simulink library "seb"  (Simulink 8.1)
settings: Solver=ode1  StartTime=0.0  StopTime=Inf  FixedStep=0.001  RelTol=1e-3
PostLoadFcn:
  | , if any(exist('dsrtsu_mdlpostloadfcn', 'file') == [2, 3, 6]), try dsrtsu_mdlpostloadfcn('Execute', bdroot); catch fprintf('Error in PostLoadFcn (dsrtsu_mdlpostloadfcn) for model "%s":\n %s\n', bdroot, lasterr); end, end,
undefined symbols (not defined in the file or in its folder): ENUM_AEBSTATE_AUTOBRAKING, ENUM_AEBSTATE_BRAKEASSIST, ENUM_AEBSTATE_DISABLED, ENUM_AEBSTATE_OPERATIONAL, ENUM_AEBSTATE_PREBRAKING, ENUM_AEBSTATE_STANDBY, ENUM_HMISTATE_ACTIVE, ENUM_HMISTATE_DISABLED, ENUM_HMISTATE_STANDBY, FALSE, TRUE, ZERO_FLOAT
settings Model: DSRTSU_INTERNAL_RTI_VER=450  DSRTSU_INTERNAL_RTI_TYPE=rti1401  RTICANMMDATA=struct('GeneralSetupData',struct('modelroot','D:\Soichi\SVNDATA\IDIADA_ADAS\trunk\AdasDragon\software\sw_development\arch\app\aeb','generalsettings',struct('filesettings',struct('destfolder',struct('Name','RTICANMM_FILES','Check',1),'buildfolder',struct('Name','.','Check',1),'AbsDestfolder',struct('Name','D:\Soichi\SVNDATA\IDIADA_ADAS\trunk\AdasDragon\software\sw_development\arch\app\aeb\RTICANMM_FILES'),'AbsBuildfolder',struct('Name','D:\Soichi\SVNDATA\IDIADA_ADAS\trunk\AdasDragon\software\sw_development\arch\app\aeb'))),'options',struct('addpaths',1,'rmpaths',1,'addtrcexclusion',logical(1),'cannavigator',struct('checkmonitoring',0),'show_usrtrc',0,'use_usrtrc',0),'advanced',struct('options',[1 1 1 1 1 1 1 1 1 1 1 1 1 1 1 1 1 1 1 1 1 1 1 1 1 1 1 1 1 1 1 1 1 1 1 1 1 1 1 1 1 1 1 1 1 1 1 1 1 1 1 1 1 1 1 1 1 1 1 1 1 1 1 1 1 1 1 1 1 1 1 1 1 1 1 1 1 1 1 1 1 1 1 1 1 1 1 1 1 1 1 1 1 1 1 1 1 1 1 1]),'MPSetup',{{}},'modelname','seb','block','seb'))  DSRTSU_INTERNAL_RTIFPGA=40  Creator=tescamilla  LastModifiedBy=AT015411

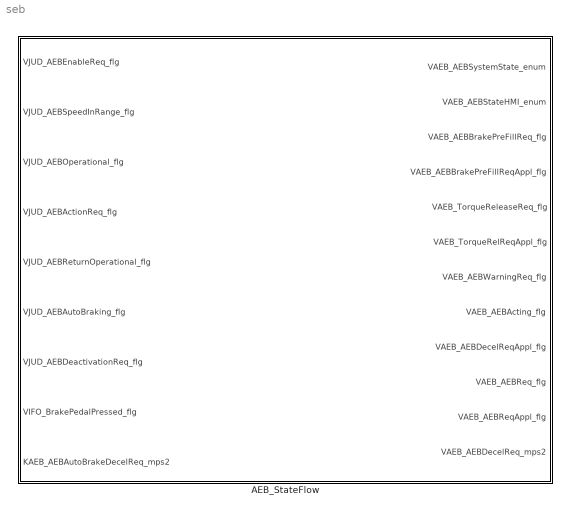
== system seb ==
  AEB_StateFlow : Stateflow chart  TreatAsAtomicUnit=on

== stateflow chart AEB_StateFlow ==
  state DISABLED
    en:
    VAEB_AEBSystemState_enum= ENUM_AEBSTATE_DISABLED;
    VAEB_AEBStateHMI_enum = ENUM_HMISTATE_DISABLED;
    VAEB_AEBWarningReq_flg = FALSE;
    VAEB_AEBActing_flg = FALSE;
    VAEB_TorqueReleaseReq_flg = FALSE;
    VAEB_TorqueRelReqAppl_flg = FALSE;
    VAEB_AEBBrakePreFillReq_flg = FALSE;
    VAEB_AEBBrakePreFillReqAppl_flg = FALSE;
    VAEB_AEBDecelReq_mps2 = ZERO_FLOAT;
    VAEB_AEBDecelReqAppl_flg = FALSE;
    VAEB_AEBReq_flg = FALSE;
    VAEB_AEBReqAppl_flg = FALSE;
  state ENABLED
    state STANDBY
      en:
      VAEB_AEBSystemState_enum = ENUM_AEBSTATE_STANDBY;
      VAEB_AEBStateHMI_enum = ENUM_HMISTATE_STANDBY;
    state ACTIVE
      state OPERATIONAL
        en:
        VAEB_AEBSystemState_enum = ENUM_AEBSTATE_OPERATIONAL;
        VAEB_AEBStateHMI_enum = ENUM_HMISTATE_STANDBY;
      state ACTING
        en:
        VAEB_AEBStateHMI_enum = ENUM_HMISTATE_ACTIVE;
        VAEB_AEBWarningReq_flg = TRUE;
        VAEB_AEBActing_flg=TRUE;
        VAEB_TorqueReleaseReq_flg = TRUE;
        VAEB_TorqueRelReqAppl_flg = TRUE;
        ex:
        VAEB_AEBWarningReq_flg = FALSE;
        VAEB_AEBActing_flg = FALSE;
        VAEB_TorqueReleaseReq_flg = FALSE;
        VAEB_TorqueRelReqAppl_flg = FALSE;
        state PREBRAKING
          en:
          VAEB_AEBSystemState_enum = ENUM_AEBSTATE_PREBRAKING;
          VAEB_AEBBrakePreFillReq_flg = TRUE;
          VAEB_AEBBrakePreFillReqAppl_flg = TRUE;
          ex:
          VAEB_AEBBrakePreFillReq_flg = FALSE;
          VAEB_AEBBrakePreFillReqAppl_flg = FALSE;
        state AUTO_BRAKING
          en:
          VAEB_AEBSystemState_enum = ENUM_AEBSTATE_AUTOBRAKING;
          VAEB_AEBDecelReqAppl_flg = TRUE;
          VAEB_AEBDecelReq_mps2 = KAEB_AEBAutoBrakeDecelReq_mps2;
          ex:
          VAEB_AEBDecelReqAppl_flg = FALSE;
          VAEB_AEBDecelReq_mps2 = ZERO_FLOAT;
        state BRAKE_ASSIST
          en:
          VAEB_AEBSystemState_enum = ENUM_AEBSTATE_BRAKEASSIST;
          VAEB_AEBReq_flg = TRUE;
          VAEB_AEBReqAppl_flg = TRUE;
          ex:
          VAEB_AEBReq_flg = FALSE;
          VAEB_AEBReqAppl_flg = FALSE;
        (default) -> PREBRAKING
        AUTO_BRAKING -> BRAKE_ASSIST : [VIFO_BrakePedalPressed_flg == TRUE]
        PREBRAKING -> AUTO_BRAKING [order 1] : [VJUD_AEBAutoBraking_flg==TRUE]
        PREBRAKING -> (junction 19) [order 2]
        (junction 20) -> BRAKE_ASSIST
        (junction 19) -> (junction 20) : [VIFO_BrakePedalPressed_flg == TRUE]
      (default) -> OPERATIONAL
      OPERATIONAL -> ACTING [order 2] : [VJUD_AEBActionReq_flg==TRUE]
      ACTING -> OPERATIONAL : [VJUD_AEBReturnOperational_flg==TRUE]
    (default) -> STANDBY
    STANDBY -> ACTIVE : [VJUD_AEBOperational_flg == TRUE]
    OPERATIONAL -> STANDBY [order 1] : [VJUD_AEBSpeedInRange_flg == FALSE]
    ACTIVE -> STANDBY : [VJUD_AEBDeactivationReq_flg==TRUE]
  (default) -> DISABLED
  DISABLED -> ENABLED : [VJUD_AEBEnableReq_flg==TRUE]
  ENABLED -> DISABLED : [VJUD_AEBEnableReq_flg==FALSE]
  data: VJUD_AEBEnableReq_flg input double; VJUD_AEBSpeedInRange_flg input double; VJUD_AEBOperational_flg input double; VJUD_AEBActionReq_flg input double; VJUD_AEBReturnOperational_flg input double; VJUD_AEBAutoBraking_flg input double; VJUD_AEBDeactivationReq_flg input double; VAEB_AEBSystemState_enum output uint8; ENUM_AEBSTATE_DISABLED parameter uint8 =0; ENUM_HMISTATE_DISABLED parameter uint8 =3; ENUM_AEBSTATE_OPERATIONAL parameter uint8 =2; ENUM_AEBSTATE_PREBRAKING parameter uint8 =3; ENUM_AEBSTATE_AUTOBRAKING parameter uint8 =4; VAEB_AEBStateHMI_enum output uint8; VAEB_AEBBrakePreFillReq_flg output boolean; VAEB_AEBBrakePreFillReqAppl_flg output boolean; VAEB_TorqueReleaseReq_flg output boolean; VAEB_TorqueRelReqAppl_flg output double; VAEB_AEBWarningReq_flg output boolean; ENUM_HMISTATE_STANDBY parameter uint8 =2; ENUM_HMISTATE_ACTIVE parameter uint8; VAEB_AEBActing_flg output boolean; VAEB_AEBDecelReqAppl_flg output boolean; FALSE parameter double; TRUE parameter double; ENUM_AEBSTATE_STANDBY parameter uint8; VIFO_BrakePedalPressed_flg input boolean; VAEB_AEBReq_flg output boolean; ENUM_AEBSTATE_BRAKEASSIST parameter uint8; VAEB_AEBReqAppl_flg output boolean; VAEB_AEBDecelReq_mps2 output single; ZERO_FLOAT parameter single; KAEB_AEBAutoBrakeDecelReq_mps2 input single
